simulink model "AFU_20b_Receive"  (R2020b)
settings: Solver=FixedStepDiscrete  StartTime=0.0  StopTime=Inf  FixedStep=1/100  RelTol=1e-3
libraries: etargetslib x2, simulink x1, slrealtimeiplib x1
settings Model: EnablePacing=on  Creator=afuzunkaya  LastModifiedBy=afuzunkaya
settings DataIOCC: ReturnWorkspaceOutputsName=Receive

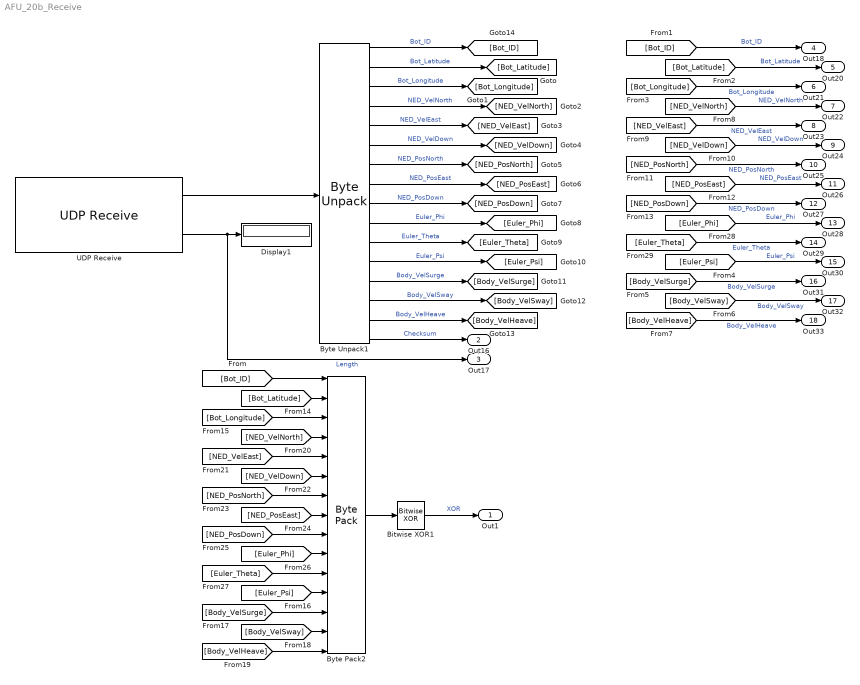
== system AFU_20b_Receive ==
  Bitwise XOR1 : simulink/Logic and Bit Operations/Bitwise Operator  logicop=XOR  UseBitMask=off  BitMask=bin2dec('11011001')  BitMaskRealWorld=Stored Integer
  Byte Pack2 : etargetslib/Byte Pack  datatypes={'uint8','int32','int32','int16','int16','int16','int32','int32','int32','int16','int16','int16','int16','int16','int16'}  byteAlign=1
  Byte Unpack1 : etargetslib/Byte Unpack  dimensions={[1],[1],[1],[1],[1],[1],[1],[1],[1],[1],[1],[1],[1],[1],[1],[1]}  datatypes={'uint8','int32','int32','int16','int16','int16','int32','int32','int32','int16','int16','int16','int16','int16','int16','uint8'}  byteAlign=1
  Display1 : Display
  UDP Receive : slrealtimeiplib/UDP Receive  useHostTargetConn=off  ipAddress=192.168.7.7  localPort=22333  rcvWidth=40  rcvFmAny=off  fmAddress=192.168.7.2  rcvMulticast=off  multicastAddress={}  sampleTime=0.1
      settings: SourceProductBaseCode=XP
  Out1 : Outport
  Out16 : Outport  Port=2
  Out17 : Outport  Port=3
  Out18 : Outport  Port=4
  Out20 : Outport  Port=5
  Out21 : Outport  Port=6
  Out22 : Outport  Port=7
  Out23 : Outport  Port=8
  Out24 : Outport  Port=9
  Out25 : Outport  Port=10
  Out26 : Outport  Port=11
  Out27 : Outport  Port=12
  Out28 : Outport  Port=13
  Out29 : Outport  Port=14
  Out30 : Outport  Port=15
  Out31 : Outport  Port=16
  Out32 : Outport  Port=17
  Out33 : Outport  Port=18
  wires:
  Byte Unpack1/15 -> [Body_VelHeave]  "Body_VelHeave"
  Byte Unpack1/5 -> [NED_VelEast]  "NED_VelEast"
  Byte Unpack1/14 -> [Body_VelSway]  "Body_VelSway"
  Byte Unpack1/12 -> [Euler_Psi]  "Euler_Psi"
  Byte Unpack1/7 -> [NED_PosNorth]  "NED_PosNorth"
  Byte Unpack1/10 -> [Euler_Phi]  "Euler_Phi"
  Byte Unpack1/3 -> [Bot_Longitude]  "Bot_Longitude"
  Byte Unpack1/13 -> [Body_VelSurge]  "Body_VelSurge"
  Byte Unpack1/6 -> [NED_VelDown]  "NED_VelDown"
  Byte Unpack1/9 -> [NED_PosDown]  "NED_PosDown"
  Byte Unpack1/4 -> [NED_VelNorth]  "NED_VelNorth"
  Byte Unpack1/16 -> Out16/1  "Checksum"
  Byte Unpack1/8 -> [NED_PosEast]  "NED_PosEast"
  Byte Unpack1/11 -> [Euler_Theta]  "Euler_Theta"
  Byte Unpack1/2 -> [Bot_Latitude]  "Bot_Latitude"
  UDP Receive/2 -> Display1/1, Out17/1  "Length"
  UDP Receive/1 -> Byte Unpack1/1
  Byte Unpack1/1 -> [Bot_ID]  "Bot_ID"
  [NED_PosDown] -> Byte Pack2/9
  [Euler_Theta] -> Byte Pack2/11
  [Body_VelSway] -> Byte Pack2/14
  [Euler_Phi] -> Byte Pack2/10
  [Body_VelHeave] -> Byte Pack2/15
  [Euler_Psi] -> Byte Pack2/12
  [NED_VelDown] -> Byte Pack2/6
  Bitwise XOR1/1 -> Out1/1  "XOR"
  [Bot_Longitude] -> Byte Pack2/3
  [NED_PosEast] -> Byte Pack2/8
  [Body_VelSurge] -> Byte Pack2/13
  [NED_VelNorth] -> Byte Pack2/4
  [NED_PosNorth] -> Byte Pack2/7
  [Bot_Latitude] -> Byte Pack2/2
  [NED_VelEast] -> Byte Pack2/5
  Byte Pack2/1 -> Bitwise XOR1/1
  [Bot_ID] -> Byte Pack2/1
  [Euler_Theta] -> Out29/1  "Euler_Theta"
  [Bot_Longitude] -> Out21/1  "Bot_Longitude"
  [Bot_ID] -> Out18/1  "Bot_ID"
  [NED_PosDown] -> Out27/1  "NED_PosDown"
  [Body_VelHeave] -> Out33/1  "Body_VelHeave"
  [NED_PosNorth] -> Out25/1  "NED_PosNorth"
  [Euler_Psi] -> Out30/1  "Euler_Psi"
  [NED_PosEast] -> Out26/1  "NED_PosEast"
  [NED_VelEast] -> Out23/1  "NED_VelEast"
  [Bot_Latitude] -> Out20/1  "Bot_Latitude"
  [Euler_Phi] -> Out28/1  "Euler_Phi"
  [NED_VelNorth] -> Out22/1  "NED_VelNorth"
  [NED_VelDown] -> Out24/1  "NED_VelDown"
  [Body_VelSway] -> Out32/1  "Body_VelSway"
  [Body_VelSurge] -> Out31/1  "Body_VelSurge"
